simulink model "Clab5"  (R2019b)
settings: Solver=VariableStepAuto  StartTime=0.0  StopTime=100  RelTol=1e-9
values from neighbouring files (symbols this model uses):
  A0 = 4E-10    (= 4e-10)    [CLAB5.m]
  B0 = 900/I0    (= 3.91304347826e-11)    [CLAB5.m]
  f = 10    [CLAB5.m]
  I0 = I/(10^i)    [CLAB5.m]
  I1 = 2.3E9    (= 2300000000)    [CLAB5.m]
  t1 = 46/1000    (= 0.046)    [CLAB5.m]
  t1b = 12.7/1000    (= 0.0127)    [CLAB5.m]
  t2 = 5.4/1000    (= 0.0054)    [CLAB5.m]
  t2b = 6.8/1000    (= 0.0068)    [CLAB5.m]
  t3 = .4/1000    (= 0.0004)    [CLAB5.m]
  t4 = 76.3/1000    (= 0.0763)    [CLAB5.m]
settings Model: Creator=PranavM  LastModifiedBy=PranavM

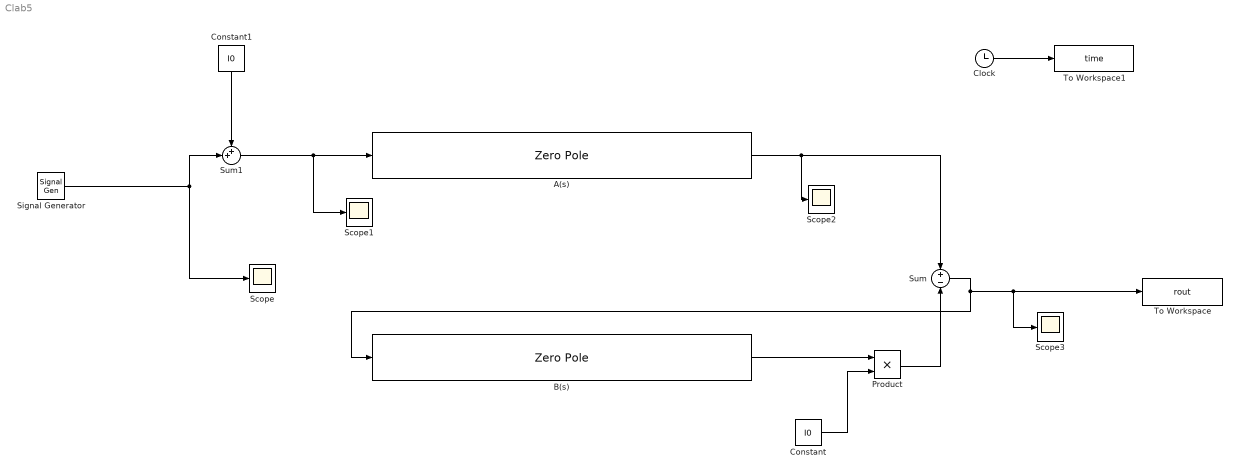
== system Clab5 ==
  A(s) : ZeroPole  Zeros=[]  Poles=[(-1/t1) (-1/t1) (-1/t1) (-1/t2) (-1/t2) (-1/t2) (-1/t2) (-1/t2) (-1/t2) (-1/t2)]  Gain=[(A0)/(((t1)^3) * ((t2)^7))]
  B(s) : ZeroPole  Zeros=[(-1/t1b) (-1/t2b) (-1/t2b) (-1/t2b)]  Poles=[(-1/t3) (-1/t4) (-1/t4) (-1/t4)]  Gain=[(B0 * t1b * ((t2b)^3))/(t3*((t4)^3))]
  Clock : Clock
  Constant : Constant  Value=I0
  Constant1 : Constant  Value=I0
  Product : Product
  Scope{,1..3} (4 alike) : Scope
  Signal Generator : SignalGenerator  Amplitude=I1  Frequency=2*pi*f  Units=rad/sec
  Sum : Sum  Inputs=+|-
  Sum1 : Sum  Inputs=++|
  To Workspace : ToWorkspace  VariableName=rout  SampleTime=-1
  To Workspace1 : ToWorkspace  VariableName=time  SampleTime=-1
  wires:
  A(s)/1 -> Scope2/1, Sum/1
  B(s)/1 -> Product/1
  Product/1 -> Sum/2
  Constant/1 -> Product/2
  Sum/1 -> Scope3/1, To Workspace/1, B(s)/1
  Constant1/1 -> Sum1/1
  Signal Generator/1 -> Sum1/2, Scope/1
  Sum1/1 -> Scope1/1, A(s)/1
  Clock/1 -> To Workspace1/1
